simulink model "udp_com"  (R2018a)
settings: Solver=VariableStepAuto  StartTime=0.0  StopTime=10  RelTol=1e-3
libraries: dspnetwork x2, sldrtlib x1
settings Model: Creator=cihad  LastModifiedBy=Cihad

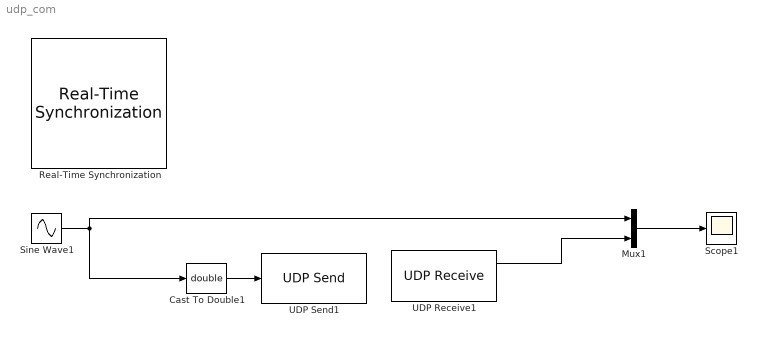
== system udp_com ==
  Cast To Double1 : DataTypeConversion  OutDataTypeStr=double
  Mux1 : Mux  Inputs=2
  Real-Time Synchronization : sldrtlib/Real-Time Synchronization  SampleTime=0.01  MaxMissedTicks=100000  ShowMissedTicks=off  YieldWhenWaiting=off
  Scope1 : Scope
  Sine Wave1 : Sin  SampleTime=0.01
  UDP Receive1 : dspnetwork/UDP Receive  localURL='0.0.0.0'  localPort=26000  remoteURL='0.0.0.0'  remotePort=-1  recvBufferSize=8192  dims=1  signalDatatype=double  isVarSize=off  showBlockingTime=off  blockingTime=0  sampletime=0.001  blockPlatform=[]
      settings: SourceProductName=DSP System Toolbox  SourceProductBaseCode=DS
  UDP Send1 : dspnetwork/UDP Send  remoteURL='127.0.0.1'  remotePort=25000  localURL='0.0.0.0'  localPortSource=Automatically determine  localPort=-1  sampletime=-1  blockPlatform=[]  separateLengthPort=0
      settings: SourceProductName=DSP System Toolbox  SourceProductBaseCode=DS
  wires:
  Mux1/1 -> Scope1/1
  Sine Wave1/1 -> Mux1/1, Cast To Double1/1
  UDP Receive1/1 -> Mux1/2
  Cast To Double1/1 -> UDP Send1/1
